simulink model "TVModel_Simulation_21"  (R2021b)
settings: Solver=FixedStepDiscrete  StartTime=0.0  StopTime=250  FixedStep=0.02  MaxStep=0.01  RelTol=1e-3
undefined symbols (not defined in the file or in its folder): MB, TV, TV_OLD
libraries: simulink x22, simulink_extras x14, eeGeneralControl x13, slpidlib x8, fuzblock x4, controlLib x4, cstblocks x3, dspstat3 x2, eeSlidingModeController x1, sharedTrackingLibrary x1
(part 4 of 9)

== system TVModel_Simulation_21/Subsystem/Subsystem1/Torque Distribution/MPC/States Constraints ==
  In Bus Element16 : Inport  PortName=torque_limits  Element=t_limit_negative
  In Bus Element3 : Inport  PortName=torque_limits  Element=t_limit_positive
  In Bus Element6 : Inport  Port=2  PortName=TC_Torque  Element=Regen
  In Bus Element7 : Inport  Port=2  PortName=TC_Torque  Element=Traction
  In Bus Element1 : Inport  Port=3  PortName=dynamics_data
  In Bus Element4 : Inport  Port=4  PortName=slip_ratio
  In Bus Element13 : Inport  Port=5  PortName=brake_signal
  In Bus Element5 : Inport  Port=6  PortName=driver_inputs  Element=brake
  In Bus Element19 : Inport  Port=6  PortName=driver_inputs  Element=throttle
  Bus Element In1 : Inport  Port=7  PortName=slip_angles
  Bus Element In11 : Inport  Port=8  PortName=Fz
  Bus Element In : Inport  Port=9  PortName=epsilon
  Anti reverse wheelspin : Subsystem
  Brake & ESP : Subsystem
  Cross Check : MATLAB Function  TreatAsAtomicUnit=on
  Low YRD : Subsystem
  MATLAB Function : MATLAB Function  TreatAsAtomicUnit=on
  MATLAB Function1 : MATLAB Function  TreatAsAtomicUnit=on
  Min : MinMax  Inputs=3
  Min1 : MinMax  Function=max  Inputs=3
  Tire Bounds : Subsystem
      settings: PortSchema="{\"entries\":[{\"content\":{\"sides\":[{\"content\":{\"connectorIds\":[\"In1\",\"In2\",\"In3\"]},\"type\":\"ConnectorPlacement.EquallySpacedRectSide\",\"uuid\":\"c905e0d5-9d26-4c00-bd7e-07ee0633c160\"},{\"content\":{\"connectorIds\":[\"Out1\",\"Out2\"],\"side\":\"RIGHT\"},\"type\":\"ConnectorPlacement.EquallySpacedRectSide\",\"uuid\":\"37cd4095-0f8c-481f-b8de-23350fc0b3e2\"},{\"content\":{\"connectorIds\":[\"Out3\"],\"side\":\"TOP\"},\"type\":\"ConnectorPlacement.EquallySpacedRectSide\",\"uuid\":\"585cff9f-4d8e-4579-999e-dff949f4791c\"}]},\"type\":\"ConnectorPlacement.EquallySpacedConnector\",\"uuid\":\"48494429-6ae2-4bc0-abe5-17d5f904d891\"}],\"packageUris\":[\"http://schema.mathworks.com/mf0/Connector/R2020b\"],\"version\":\"1.0\"}"
  Unary Minus : UnaryMinus
  lbx : Outport
  ubx : Outport  Port=2
  Out Bus Element2 : Outport  Port=3  PortName=TV_Info  Element=ubx
  Out Bus Element3 : Outport  Port=3  PortName=TV_Info  Element=lbx
  Out Bus Element1 : Outport  Port=3  PortName=TV_Info  Element=Tire_Bounds
  wires:
  In Bus Element19/1 -> Cross Check/5(throttle)
  Bus Element In/1 -> Cross Check/4(epsilon)
  In Bus Element7/1 -> Min/2
  Min1/1 -> Anti reverse wheelspin/1(lbx_in), Low YRD/2(lbx_max)
  Low YRD/1(bounds) -> Cross Check/2(bounds)
  Anti reverse wheelspin/1(lbx_out) -> Cross Check/3(lbx_in), Low YRD/3(lbx_in)
  MATLAB Function1/1(y) -> lbx/1
  MATLAB Function/1(y) -> ubx/1
  In Bus Element16/1 -> Unary Minus/1
  Cross Check/1(ubx_out) -> Out Bus Element2/1, MATLAB Function/1(u)
  Bus Element In1/1 -> Tire Bounds/2(slip_angle)
  Bus Element In11/1 -> Tire Bounds/1(fz)
  Tire Bounds/3(TV_Info) -> Out Bus Element1/1
  In Bus Element1/1 -> Tire Bounds/3(dynamics_data)
  Tire Bounds/1(tire_ubx) -> Min/3
  Tire Bounds/2(tire_lbx) -> Min1/1
  Min/1 -> Brake & ESP/1(ubx_in)
  Brake & ESP/1(ubx_out) -> Cross Check/1(ubx_in), Low YRD/1(ubx_in)
  In Bus Element13/1 -> Brake & ESP/2(brake_signal)
  In Bus Element4/1 -> Anti reverse wheelspin/2(slip_ratio)
  In Bus Element5/1 -> Cross Check/6(brake)
  In Bus Element6/1 -> Min1/3
  In Bus Element3/1 -> Min/1
  Unary Minus/1 -> Min1/2
  Cross Check/2(lbx_out) -> MATLAB Function1/1(u), Out Bus Element3/1

== system TVModel_Simulation_21/Subsystem/Subsystem1/Torque Distribution/MPC/USEFUL STUFFFF ==
  In Bus Element10 : Inport  PortName=front_wheels_steering  Element=single_axis
  Abs : Abs  Commented=on
  Chart : Stateflow chart  Commented=on  TreatAsAtomicUnit=on
  Constant3 : Constant  Commented=on  Value=TV.SIGNALS.SETTINGS.steer_threshold
  Constant5 : Constant  Commented=on  Value=TV.SIGNALS.SETTINGS.steer_relay_amplitude
  Extended Kalman Filter : Subsystem  Commented=on
  Non-Linear Activation : MATLAB Function  Commented=on  TreatAsAtomicUnit=on
  Power Limiter : Subsystem  Commented=on
  Power flag : Subsystem  Commented=on
  Radians to Degrees : simulink_extras/Transformations/Radians to Degrees  Commented=on
  States Selector : Subsystem  Commented=on
  Subsystem : Subsystem  Commented=on
  Subsystem1 : Subsystem  Commented=on
  Yrd 0 When Steering 0 : Subsystem  Commented=on
      mask Display: image('Mask_Icon\On_Off.png'); % Use "Edit Image" on toolstrip to change.
  lbu_dot : Subsystem  Commented=on
  wires:
  Power flag/1(Output) -> ?
  Subsystem/1(Output) -> ?
  Abs/1 -> Chart/1(front_wheels_steering)
  In Bus Element10/1 -> Radians to Degrees/1
  Constant5/1 -> Chart/2(semi_amplitude)
  Radians to Degrees/1 -> Abs/1
  Constant3/1 -> Chart/3(steer_threshold)

== system TVModel_Simulation_21/Subsystem/Subsystem1/Torque Distribution/MPC/Useful Calculations ==
  In Bus Element16 : Inport  PortName=dynamics_data
  In Bus Element1 : Inport  PortName=dynamics_data  Element=omega_wheels
  In Bus Element18 : Inport  Port=2  PortName=front_wheel_angles  Element=different_axis
  Inport : Inport  Port=3
  Abs : Abs
  Gain : Gain  Gain=13.5
  Inport1 : InportShadow  Port=3
  MATLAB Function : MATLAB Function  TreatAsAtomicUnit=on
  MATLAB Function1 : MATLAB Function  TreatAsAtomicUnit=on
  MATLAB Function2 : MATLAB Function  TreatAsAtomicUnit=on
  Power Calculation Post : Subsystem
  Terminator{,1..3} (4 alike) : Terminator
  wires:
  Abs/1 -> MATLAB Function2/2(t)
  Gain/1 -> MATLAB Function2/1(omega)
  In Bus Element1/1 -> Gain/1
  MATLAB Function2/1(y) -> Terminator3/1  "p_MPC"
  MATLAB Function1/2(deltag4) -> Terminator2/1  "deltag4"
  MATLAB Function1/1(deltag3) -> Terminator1/1  "deltag3"
  Inport1/1 -> MATLAB Function/1(T), MATLAB Function1/1(u), Abs/1
  Inport/1 -> Power Calculation Post/2(Motor_Torque)
  In Bus Element18/1 -> MATLAB Function/2(delta)
  MATLAB Function/1(y) -> Terminator/1  "Mz_Real"
  In Bus Element16/1 -> Power Calculation Post/1(dynamics_data)

== system TVModel_Simulation_21/Subsystem/Subsystem1/Torque Distribution/MPC/Weights Generation ==
  In Bus Element1 : Inport  PortName=dynamics_data
  Torque : Inport  Port=2
  Constant : Constant  Value=1e-5*ones(4,1)
  Constant1 : Constant  Value=0  VectorParams1D=off
  Constant2 : Constant  Value=1e-4*ones(4,1)
  Demux : Demux
  Demux1 : Demux
  Efficiency limit : Subsystem  Commented=on
  Gain : Gain  Commented=on  Gain=TV.SIGNALS.SETTINGS.TorqueWeight
  MATLAB Function : MATLAB Function  TreatAsAtomicUnit=on
  Mux : Mux  Inputs=TV.MPC.ny
  r1 : Constant
  vx : Constant  Value=0
  vy : Constant  Value=TV.SIGNALS.SETTINGS.VyWeight
  w : Outport
  Out Bus Element3 : Outport  Port=2  PortName=TV_Info  Element=w
  wires:
  Constant2/1 -> Demux/1
  Efficiency limit/1(efficiency_limit) -> Gain/1
  Constant/1 -> Demux1/1
  Demux1/2 -> Mux/9
  Demux1/4 -> Mux/11
  Demux1/1 -> Mux/8
  Demux1/3 -> Mux/10
  vy/1 -> Mux/2
  vx/1 -> Mux/1
  MATLAB Function/1(y) -> Out Bus Element3/1, w/1
  Demux/1 -> Mux/4
  Demux/2 -> Mux/5
  Demux/4 -> Mux/7
  Demux/3 -> Mux/6
  Torque/1 -> Efficiency limit/1(motor_torque)
  In Bus Element1/1 -> Efficiency limit/2(dynamics_data)
  r1/1 -> Mux/3
  Constant1/1 -> MATLAB Function/2(deltaAxle)
  Mux/1 -> MATLAB Function/1(u)

== system TVModel_Simulation_21/Subsystem/Subsystem1/Torque Distribution/Reference Tracking/YRD_LUT_-1 ==
  front_wheel_angle : Inport
  vx : Inport  Port=2
  Action Port : ActionPort  ActionPortLabel=elseif(u1 ==4)
  Abs : Abs
  Cast3 : DataTypeConversion  Commented=on  OutDataTypeStr=single
  Divide : Product  Inputs=*/
  Divide1 : Product  Inputs=*/
  Divide2 : Product  Inputs=**
  LUT_-3 : Lookup_n-D  BreakpointsForDimension1=TV.LUT.Yrd_LUT.LUT_vectors.delta_vector  BreakpointsForDimension2=TV.LUT.Yrd_LUT.LUT_vectors.v_vector  Table=single(TV.LUT.Yrd_LUT.LUT_neg3.ay_matrix)  InternalRulePriority=Speed  RndMeth=Simplest  InputSameDT=on
      settings: InputPortMap=u0,u1
  Saturation : Saturate  UpperLimit=inf  LowerLimit=3
  yrd : Outport
  wires:
  Divide1/1 -> Divide2/1  "normalized_front_wheel_angle"
  Divide2/1 -> yrd/1  "yrd"
  Saturation/1 -> LUT_-3/2, Divide/2  "vx"
  vx/1 -> Saturation/1
  LUT_-3/1 -> Divide/1  "a"
  Divide/1 -> Divide2/2
  Abs/1 -> LUT_-3/1, Divide1/2  "absolute_front_wheel_angle"
  front_wheel_angle/1 -> Abs/1, Divide1/1

== system TVModel_Simulation_21/Subsystem/Subsystem1/Torque Distribution/Reference Tracking/YRD_LUT_-1.1 ==
  front_wheel_angle : Inport
  vx : Inport  Port=2
  Action Port : ActionPort  ActionPortLabel=elseif(u1 ==3)
  Abs : Abs
  Cast3 : DataTypeConversion  Commented=on  OutDataTypeStr=single
  Divide : Product  Inputs=*/
  Divide1 : Product  Inputs=*/
  Divide2 : Product  Inputs=**
  LUT_-1.5 : Lookup_n-D  BreakpointsForDimension1=TV.LUT.Yrd_LUT.LUT_vectors.delta_vector  BreakpointsForDimension2=TV.LUT.Yrd_LUT.LUT_vectors.v_vector  Table=single(TV.LUT.Yrd_LUT.LUT_neg1_5.ay_matrix)  InternalRulePriority=Speed  RndMeth=Simplest  InputSameDT=on
      settings: InputPortMap=u0,u1
  Saturation : Saturate  UpperLimit=inf  LowerLimit=3
  yrd : Outport
  wires:
  Divide/1 -> Divide2/2
  LUT_-1.5/1 -> Divide/1
  Saturation/1 -> LUT_-1.5/2, Divide/2  "vx"
  Abs/1 -> LUT_-1.5/1, Divide1/2  "absolute_front_wheel_angle"
  Divide2/1 -> yrd/1  "yrd"
  Divide1/1 -> Divide2/1  "normalized_front_wheel_angle"
  vx/1 -> Saturation/1
  front_wheel_angle/1 -> Abs/1, Divide1/1

== system TVModel_Simulation_21/Subsystem/Subsystem1/Torque Distribution/Reference Tracking/YRD_LUT_-1.5 ==
  front_wheel_angle : Inport
  vx : Inport  Port=2
  Action Port : ActionPort  ActionPortLabel=elseif(u1 ==3)
  Abs : Abs
  Cast3 : DataTypeConversion  Commented=on  OutDataTypeStr=single
  Divide : Product  Inputs=*/
  Divide1 : Product  Inputs=*/
  Divide2 : Product  Inputs=**
  LUT_-1.5 : Lookup_n-D  BreakpointsForDimension1=TV.LUT.Yrd_LUT.LUT_vectors.delta_vector  BreakpointsForDimension2=TV.LUT.Yrd_LUT.LUT_vectors.v_vector  Table=single(TV.LUT.Yrd_LUT.LUT_neg1_5.ay_matrix)  InternalRulePriority=Speed  RndMeth=Simplest  InputSameDT=on
      settings: InputPortMap=u0,u1
  Saturation : Saturate  UpperLimit=inf  LowerLimit=3
  yrd : Outport
  wires:
  front_wheel_angle/1 -> Divide1/1, Abs/1
  vx/1 -> Saturation/1
  Divide1/1 -> Divide2/1  "normalized_front_wheel_angle"
  Divide2/1 -> yrd/1  "yrd"
  Abs/1 -> Divide1/2, LUT_-1.5/1  "absolute_front_wheel_angle"
  Saturation/1 -> Divide/2, LUT_-1.5/2  "vx"
  LUT_-1.5/1 -> Divide/1
  Divide/1 -> Divide2/2

== system TVModel_Simulation_21/Subsystem/Subsystem1/Torque Distribution/Reference Tracking/YRD_LUT_-3 ==
  front_wheel_angle : Inport
  vx : Inport  Port=2
  Action Port : ActionPort  ActionPortLabel=elseif(u1 ==4)
  Abs : Abs
  Cast3 : DataTypeConversion  Commented=on  OutDataTypeStr=single
  Divide : Product  Inputs=*/
  Divide1 : Product  Inputs=*/
  Divide2 : Product  Inputs=**
  LUT_-3 : Lookup_n-D  BreakpointsForDimension1=TV.LUT.Yrd_LUT.LUT_vectors.delta_vector  BreakpointsForDimension2=TV.LUT.Yrd_LUT.LUT_vectors.v_vector  Table=single(TV.LUT.Yrd_LUT.LUT_neg3.ay_matrix)  InternalRulePriority=Speed  RndMeth=Simplest  InputSameDT=on
      settings: InputPortMap=u0,u1
  Saturation : Saturate  UpperLimit=inf  LowerLimit=3
  yrd : Outport
  wires:
  front_wheel_angle/1 -> Divide1/1, Abs/1
  Abs/1 -> Divide1/2, LUT_-3/1  "absolute_front_wheel_angle"
  Divide/1 -> Divide2/2
  LUT_-3/1 -> Divide/1  "a"
  vx/1 -> Saturation/1
  Saturation/1 -> Divide/2, LUT_-3/2  "vx"
  Divide2/1 -> yrd/1  "yrd"
  Divide1/1 -> Divide2/1  "normalized_front_wheel_angle"

== system TVModel_Simulation_21/Subsystem/Subsystem1/Torque Distribution/Reference Tracking/YRD_LUT_0 ==
  front_wheel_angle : Inport
  vx : Inport  Port=2
  Action Port : ActionPort  ActionPortLabel=elseif(u1 ==2)
  Abs : Abs
  Cast : DataTypeConversion  Commented=on  OutDataTypeStr=single
  Divide : Product  Inputs=*/
  Divide1 : Product  Inputs=*/
  Divide2 : Product  Inputs=**
  LUT_0 : Lookup_n-D  BreakpointsForDimension1=TV.LUT.Yrd_LUT.LUT_vectors.delta_vector  BreakpointsForDimension2=TV.LUT.Yrd_LUT.LUT_vectors.v_vector  Table=single(TV.LUT.Yrd_LUT.LUT_0.ay_matrix)  InternalRulePriority=Speed  RndMeth=Simplest  InputSameDT=on
      settings: InputPortMap=u0,u1
  Saturation : Saturate  UpperLimit=inf  LowerLimit=3
  yrd : Outport
  wires:
  front_wheel_angle/1 -> Divide1/1, Abs/1
  Saturation/1 -> Divide/2, LUT_0/2  "vx"
  Abs/1 -> Divide1/2, LUT_0/1  "absolute_front_wheel_angle"
  Divide2/1 -> yrd/1  "yrd"
  vx/1 -> Saturation/1
  Divide/1 -> Divide2/2
  Divide1/1 -> Divide2/1  "normalized_front_wheel_angle"
  LUT_0/1 -> Divide/1

== system TVModel_Simulation_21/Subsystem/Subsystem1/Torque Distribution/Reference Tracking/YRD_LUT_1 ==
  front_wheel_angle : Inport
  vx : Inport  Port=2
  Action Port : ActionPort  ActionPortLabel=if(u1 == 1)
  Abs : Abs
  Cast3 : DataTypeConversion  Commented=on  OutDataTypeStr=single
  Divide : Product  Inputs=*/
  Divide1 : Product  Inputs=*/
  Divide2 : Product  Inputs=**
  LUT_1 : Lookup_n-D  BreakpointsForDimension1=TV.LUT.Yrd_LUT.LUT_vectors.delta_vector  BreakpointsForDimension2=TV.LUT.Yrd_LUT.LUT_vectors.v_vector  Table=single(TV.LUT.Yrd_LUT.LUT_1.ay_matrix)  InternalRulePriority=Speed  RndMeth=Simplest  InputSameDT=on
      settings: InputPortMap=u0,u1
  Saturation : Saturate  UpperLimit=inf  LowerLimit=3
  yrd : Outport
  wires:
  front_wheel_angle/1 -> Divide1/1, Abs/1
  LUT_1/1 -> Divide/1
  vx/1 -> Saturation/1
  Divide1/1 -> Divide2/1  "normalized_front_wheel_angle"
  Divide2/1 -> yrd/1  "yrd"
  Abs/1 -> Divide1/2, LUT_1/1  "absolute_front_wheel_angle"
  Saturation/1 -> Divide/2, LUT_1/2  "vx"
  Divide/1 -> Divide2/2

== system TVModel_Simulation_21/Subsystem/Subsystem1/Torque Distribution/Reference Tracking/YRD_LUT_2 ==
  front_wheel_angle : Inport
  vx : Inport  Port=2
  Action Port : ActionPort  ActionPortLabel=elseif(u1 ==2)
  Abs : Abs
  Cast : DataTypeConversion  Commented=on  OutDataTypeStr=single
  Divide : Product  Inputs=*/
  Divide1 : Product  Inputs=*/
  Divide2 : Product  Inputs=**
  LUT_0 : Lookup_n-D  BreakpointsForDimension1=TV.LUT.Yrd_LUT.LUT_vectors.delta_vector  BreakpointsForDimension2=TV.LUT.Yrd_LUT.LUT_vectors.v_vector  Table=single(TV.LUT.Yrd_LUT.LUT_0.ay_matrix)  InternalRulePriority=Speed  RndMeth=Simplest  InputSameDT=on
      settings: InputPortMap=u0,u1
  Saturation : Saturate  UpperLimit=inf  LowerLimit=3
  yrd : Outport
  wires:
  LUT_0/1 -> Divide/1
  Divide1/1 -> Divide2/1  "normalized_front_wheel_angle"
  Divide/1 -> Divide2/2
  vx/1 -> Saturation/1
  Divide2/1 -> yrd/1  "yrd"
  Abs/1 -> LUT_0/1, Divide1/2  "absolute_front_wheel_angle"
  Saturation/1 -> LUT_0/2, Divide/2  "vx"
  front_wheel_angle/1 -> Abs/1, Divide1/1

== system TVModel_Simulation_21/Subsystem/Subsystem1/Torque Distribution/Reference Tracking/YRD_LUT_3 ==
  front_wheel_angle : Inport
  vx : Inport  Port=2
  Action Port : ActionPort  ActionPortLabel=if(u1 == 1)
  Abs : Abs
  Cast3 : DataTypeConversion  Commented=on  OutDataTypeStr=single
  Divide : Product  Inputs=*/
  Divide1 : Product  Inputs=*/
  Divide2 : Product  Inputs=**
  LUT_1 : Lookup_n-D  BreakpointsForDimension1=TV.LUT.Yrd_LUT.LUT_vectors.delta_vector  BreakpointsForDimension2=TV.LUT.Yrd_LUT.LUT_vectors.v_vector  Table=single(TV.LUT.Yrd_LUT.LUT_1.ay_matrix)  InternalRulePriority=Speed  RndMeth=Simplest  InputSameDT=on
      settings: InputPortMap=u0,u1
  Saturation : Saturate  UpperLimit=inf  LowerLimit=3
  yrd : Outport
  wires:
  Divide/1 -> Divide2/2
  Saturation/1 -> LUT_1/2, Divide/2  "vx"
  Abs/1 -> LUT_1/1, Divide1/2  "absolute_front_wheel_angle"
  Divide2/1 -> yrd/1  "yrd"
  Divide1/1 -> Divide2/1  "normalized_front_wheel_angle"
  vx/1 -> Saturation/1
  LUT_1/1 -> Divide/1
  front_wheel_angle/1 -> Abs/1, Divide1/1

== system TVModel_Simulation_21/Subsystem/Subsystem1/Torque Limits/Torque Limits Positive/Torque_Curve ==
  omega_wheels : Inport
  voltage [ID380] : Inport  Port=2
  torque_map : Inport  Port=3
  2-D Lookup Table : Lookup_n-D  BreakpointsForDimension1=TV.LV.TORQUE.T_lim_pos.breakpoints1  BreakpointsForDimension2=TV.LV.TORQUE.T_lim_pos.breakpoints2  Table=TV.LV.TORQUE.T_lim_pos.table_data  ExtrapMethod=Clip  InternalRulePriority=Speed  OutDataTypeStr=double  RndMeth=Simplest  InputSameDT=on
      settings: InputPortMap=u0,u1
  Constant : Constant  Value=0
  Constant1 : Constant  Value=TV.LV.TORQUE.T_peak_motor
  Constant2 : Constant  Value=TV.LV.TORQUE.T_nominal_motor
  Gain : Gain  Gain=TV.LV.TORQUE.T_nominal_motor/1000
  Gain4 : Gain  Gain=TV.CAR.Tau*60/(2*pi)
  Low-Pass Filter (Discrete or Continuous) : eeGeneralControl/Low-Pass Filter (Discrete or Continuous)  K=1  T=1/4/pi  B=inf  A=-inf  init_option=Inherited from block input  x0=0  Ts=TV.MPC.T/TV.MPC.N
  Multiport Switch : MultiPortSwitch  DataPortOrder=Specify indices  DataPortIndices={TV.LV.TORQUE.T_peak_setting,TV.LV.TORQUE.T_nominal_setting}  DiagnosticForDefault=None
  Saturation Dynamic : simulink/Discontinuities/Saturation Dynamic  OutMin=[]  OutMax=[]  OutDataTypeStr=Inherit: Same as second input  OutDataType=fixdt(1, 16)  OutScaling=2^-10  DoSatur=off
  Saturation1 : Saturate  UpperLimit=+inf  LowerLimit=0
  max_torque_available : Outport
  wires:
  Low-Pass Filter (Discrete or Continuous)/1 -> Saturation Dynamic/2
  omega_wheels/1 -> Gain4/1
  Constant/1 -> Saturation Dynamic/3
  torque_map/1 -> Multiport Switch/1
  Constant1/1 -> Multiport Switch/2
  Constant2/1 -> Multiport Switch/3
  Multiport Switch/1 -> Saturation Dynamic/1  "torque map selected"
  Saturation1/1 -> 2-D Lookup Table/1
  voltage [ID380]/1 -> 2-D Lookup Table/2
  Gain/1 -> Low-Pass Filter (Discrete or Continuous)/1
  2-D Lookup Table/1 -> Gain/1
  Gain4/1 -> Saturation1/1  "RPM_Motors"
  Saturation Dynamic/1 -> max_torque_available/1

== system TVModel_Simulation_21/Subsystem/Subsystem1/Torque Limits/Torque Limits Regen/Torque_Curve ==
  omega_wheels : Inport
  voltage [ID380] : Inport  Port=2
  torque_map : Inport  Port=3
  2-D Lookup Table : Lookup_n-D  BreakpointsForDimension1=TV.LV.TORQUE.T_lim_pos.breakpoints1  BreakpointsForDimension2=TV.LV.TORQUE.T_lim_pos.breakpoints2  Table=TV.LV.TORQUE.T_lim_pos.table_data  ExtrapMethod=Clip  InternalRulePriority=Speed  OutDataTypeStr=double  RndMeth=Simplest  InputSameDT=on
      settings: InputPortMap=u0,u1
  Constant : Constant  Value=0
  Constant1 : Constant  Value=TV.LV.TORQUE.T_peak_motor
  Constant2 : Constant  Value=TV.LV.TORQUE.T_nominal_motor
  Gain : Gain  Gain=TV.LV.TORQUE.T_nominal_motor/1000
  Gain4 : Gain  Gain=TV.CAR.Tau*60/(2*pi)
  Low-Pass Filter (Discrete or Continuous) : eeGeneralControl/Low-Pass Filter (Discrete or Continuous)  K=1  T=1/4/pi  B=inf  A=-inf  init_option=Inherited from block input  x0=0  Ts=TV.MPC.T/TV.MPC.N
  Multiport Switch : MultiPortSwitch  DataPortOrder=Specify indices  DataPortIndices={TV.LV.TORQUE.T_peak_setting,TV.LV.TORQUE.T_nominal_setting}  DiagnosticForDefault=None
  Saturation Dynamic : simulink/Discontinuities/Saturation Dynamic  OutMin=[]  OutMax=[]  OutDataTypeStr=Inherit: Same as second input  OutDataType=fixdt(1, 16)  OutScaling=2^-10  DoSatur=off
  Saturation1 : Saturate  UpperLimit=+inf  LowerLimit=0
  max_torque_available : Outport
  wires:
  Low-Pass Filter (Discrete or Continuous)/1 -> Saturation Dynamic/2
  omega_wheels/1 -> Gain4/1
  Constant/1 -> Saturation Dynamic/3
  torque_map/1 -> Multiport Switch/1
  Constant1/1 -> Multiport Switch/2
  Constant2/1 -> Multiport Switch/3
  Multiport Switch/1 -> Saturation Dynamic/1  "torque map selected"
  Saturation1/1 -> 2-D Lookup Table/1
  voltage [ID380]/1 -> 2-D Lookup Table/2
  Gain/1 -> Low-Pass Filter (Discrete or Continuous)/1
  2-D Lookup Table/1 -> Gain/1
  Gain4/1 -> Saturation1/1  "RPM_Motors"
  Saturation Dynamic/1 -> max_torque_available/1

== system TVModel_Simulation_21/Subsystem/Subsystem1/Slip Control/Traction Control/ABS/Load Transfer Calculation1 ==
  In Bus Element : Inport  PortName=dynamics_data
  Fz FL : Subsystem
  Fz FR : Subsystem
  Fz RL : Subsystem
  Fz RR : Subsystem
  Mux : Mux
  Fz [4x1] : Outport
  wires:
  In Bus Element/1 -> Fz FL/1(dynamics_data), Fz FR/1(dynamics_data), Fz RL/1(dynamics_data), Fz RR/1(dynamics_data)
  Fz FL/1(TV_Info) -> Mux/1  "Fz_FL"
  Fz FR/1(TV_Info) -> Mux/2  "Fz_FR"
  Fz RL/1(TV_Info) -> Mux/3  "Fz_RL"
  Fz RR/1(TV_Info) -> Mux/4  "Fz_RR"
  Mux/1 -> Fz [4x1]/1

== system TVModel_Simulation_21/Subsystem/Subsystem1/Slip Control/Traction Control/ABS/Subsystem ==
  Inport : Inport
  Inport1 : Inport  Port=2
  Chart : Stateflow chart  TreatAsAtomicUnit=on
  Chart1 : Stateflow chart  TreatAsAtomicUnit=on
  Chart2 : Stateflow chart  TreatAsAtomicUnit=on
  Chart3 : Stateflow chart  TreatAsAtomicUnit=on
  Demux : Demux
  Demux1 : Demux
  Mux : Mux
  Output : Outport
  wires:
  Demux/1 -> Chart/2(epsilon)
  Demux/2 -> Chart1/2(epsilon)
  Demux/3 -> Chart2/2(epsilon)
  Demux/4 -> Chart3/2(epsilon)
  Demux1/4 -> Chart3/1(T_ff)
  Demux1/3 -> Chart2/1(T_ff)
  Demux1/2 -> Chart1/1(T_ff)
  Demux1/1 -> Chart/1(T_ff)
  Inport/1 -> Demux1/1
  Inport1/1 -> Demux/1
  Mux/1 -> Output/1  "TC_output"
  Chart3/1(TC_max) -> Mux/4  "TC_output"
  Chart2/1(TC_max) -> Mux/3  "TC_output"
  Chart1/1(TC_max) -> Mux/2  "TC_output"
  Chart/1(TC_max) -> Mux/1  "TC_output"

== system TVModel_Simulation_21/Subsystem/Subsystem1/Slip Control/Traction Control/Load Transfer calculation/Fz FL ==
  In Bus Element : Inport  PortName=dynamics_data  Element=ay
  In Bus Element1 : Inport  PortName=dynamics_data  Element=vx
  In Bus Element2 : Inport  PortName=dynamics_data  Element=ax
  Drag moment : Gain  Gain=0.5*TV.CAR.rho*TV.CAR.CdA*TV.CAR.hcop/TV.CAR.wb*0.5
  Lateral Load Transfer : Gain  Gain=TV.CAR.m/TV.CAR.tf*TV.CAR.hcog*0.5*0.5
  Lift Force : Gain  Gain=0.5*TV.CAR.rho*TV.CAR.ClA*(1-TV.CAR.xcop/TV.CAR.wb)*0.5
  Longitudinal Load Transfer : Gain  Gain=TV.CAR.m/TV.CAR.wb*TV.CAR.hcog*0.5
  Square1 : Math  Operator=square  SaturateOnIntegerOverflow=on
  Square2 : Math  Operator=square  SaturateOnIntegerOverflow=on
  Static Load Front : Constant  Value=TV.CAR.Fzf
  Subtract : Sum  Inputs=+++-+
  Unary Minus : UnaryMinus
  Unary Minus1 : UnaryMinus
  TV_Info : Outport
  wires:
  Unary Minus1/1 -> Longitudinal Load Transfer/1
  Unary Minus/1 -> Lateral Load Transfer/1
  In Bus Element/1 -> Unary Minus/1
  Subtract/1 -> TV_Info/1
  Drag moment/1 -> Subtract/4
  Static Load Front/1 -> Subtract/1
  Square1/1 -> Lift Force/1
  Lateral Load Transfer/1 -> Subtract/2
  Longitudinal Load Transfer/1 -> Subtract/5
  In Bus Element2/1 -> Unary Minus1/1
  Square2/1 -> Drag moment/1
  In Bus Element1/1 -> Square2/1, Square1/1
  Lift Force/1 -> Subtract/3

== system TVModel_Simulation_21/Subsystem/Subsystem1/Slip Control/Traction Control/Load Transfer calculation/Fz FR ==
  In Bus Element : Inport  PortName=dynamics_data  Element=ay
  In Bus Element1 : Inport  PortName=dynamics_data  Element=vx
  In Bus Element2 : Inport  PortName=dynamics_data  Element=ax
  Drag moment : Gain  Gain=0.5*TV.CAR.rho*TV.CAR.CdA*TV.CAR.hcop/TV.CAR.wb*0.5
  Lateral Load Transfer : Gain  Gain=TV.CAR.m/TV.CAR.tf*TV.CAR.hcog*0.5*0.5
  Lift Force : Gain  Gain=0.5*TV.CAR.rho*TV.CAR.ClA*(1 - TV.CAR.xcop/TV.CAR.wb)*0.5
  Longitudinal Load Transfer : Gain  Gain=TV.CAR.m/TV.CAR.wb*TV.CAR.hcog*0.5
  Square1 : Math  Operator=square  SaturateOnIntegerOverflow=on
  Square2 : Math  Operator=square  SaturateOnIntegerOverflow=on
  Static Load Front : Constant  Value=TV.CAR.Fzf
  Subtract : Sum  Inputs=+-+-+
  Unary Minus : UnaryMinus
  Unary Minus1 : UnaryMinus
  TV_Info : Outport
  wires:
  Unary Minus1/1 -> Longitudinal Load Transfer/1
  Unary Minus/1 -> Lateral Load Transfer/1
  Subtract/1 -> TV_Info/1
  Drag moment/1 -> Subtract/4
  In Bus Element/1 -> Unary Minus/1
  In Bus Element1/1 -> Square1/1, Square2/1
  Static Load Front/1 -> Subtract/1
  Square1/1 -> Lift Force/1
  Lateral Load Transfer/1 -> Subtract/2
  Longitudinal Load Transfer/1 -> Subtract/5
  In Bus Element2/1 -> Unary Minus1/1
  Lift Force/1 -> Subtract/3
  Square2/1 -> Drag moment/1

== system TVModel_Simulation_21/Subsystem/Subsystem1/Slip Control/Traction Control/Load Transfer calculation/Fz RL ==
  In Bus Element : Inport  PortName=dynamics_data  Element=ay
  In Bus Element1 : Inport  PortName=dynamics_data  Element=vx
  In Bus Element2 : Inport  PortName=dynamics_data  Element=ax
  Drag moment : Gain  Gain=0.5*TV.CAR.rho*TV.CAR.CdA*TV.CAR.hcop/TV.CAR.wb*0.5
  Lateral Load Transfer : Gain  Gain=TV.CAR.m/TV.CAR.tr*TV.CAR.hcog*0.5*0.5
  Lift Force : Gain  Gain=0.5*TV.CAR.rho*TV.CAR.ClA*(TV.CAR.xcop/TV.CAR.wb)*0.5
  Longitudinal Load Transfer : Gain  Gain=TV.CAR.m/TV.CAR.wb*TV.CAR.hcog*0.5
  Square1 : Math  Operator=square  SaturateOnIntegerOverflow=on
  Square2 : Math  Operator=square  SaturateOnIntegerOverflow=on
  Static Load Front : Constant  Value=TV.CAR.Fzr
  Subtract : Sum  Inputs=++++-
  Unary Minus : UnaryMinus
  Unary Minus1 : UnaryMinus
  TV_Info : Outport
  wires:
  Unary Minus1/1 -> Longitudinal Load Transfer/1
  Unary Minus/1 -> Lateral Load Transfer/1
  Subtract/1 -> TV_Info/1
  Drag moment/1 -> Subtract/4
  In Bus Element/1 -> Unary Minus/1
  Static Load Front/1 -> Subtract/1
  Square1/1 -> Lift Force/1
  Lateral Load Transfer/1 -> Subtract/2
  Longitudinal Load Transfer/1 -> Subtract/5
  In Bus Element2/1 -> Unary Minus1/1
  Lift Force/1 -> Subtract/3
  Square2/1 -> Drag moment/1
  In Bus Element1/1 -> Square2/1, Square1/1

== system TVModel_Simulation_21/Subsystem/Subsystem1/Slip Control/Traction Control/Load Transfer calculation/Fz RR ==
  In Bus Element : Inport  PortName=dynamics_data  Element=ay
  In Bus Element1 : Inport  PortName=dynamics_data  Element=vx
  In Bus Element2 : Inport  PortName=dynamics_data  Element=ax
  Drag moment : Gain  Gain=0.5*TV.CAR.rho*TV.CAR.CdA*TV.CAR.hcop/TV.CAR.wb*0.5
  Lateral Load Transfer : Gain  Gain=TV.CAR.m/TV.CAR.tr*TV.CAR.hcog*0.5*0.5
  Lift Force : Gain  Gain=0.5*TV.CAR.rho*TV.CAR.ClA*(TV.CAR.xcop/TV.CAR.wb)*0.5
  Longitudinal Load Transfer : Gain  Gain=TV.CAR.m/TV.CAR.wb*TV.CAR.hcog*0.5
  Square1 : Math  Operator=square  SaturateOnIntegerOverflow=on
  Square2 : Math  Operator=square  SaturateOnIntegerOverflow=on
  Static Load Front : Constant  Value=TV.CAR.Fzr
  Subtract : Sum  Inputs=+-++-
  Unary Minus : UnaryMinus
  Unary Minus1 : UnaryMinus
  TV_Info : Outport
  wires:
  Unary Minus1/1 -> Longitudinal Load Transfer/1
  Unary Minus/1 -> Lateral Load Transfer/1
  Subtract/1 -> TV_Info/1
  Drag moment/1 -> Subtract/4
  In Bus Element/1 -> Unary Minus/1
  In Bus Element1/1 -> Square1/1, Square2/1
  Static Load Front/1 -> Subtract/1
  Square1/1 -> Lift Force/1
  Lateral Load Transfer/1 -> Subtract/2
  Longitudinal Load Transfer/1 -> Subtract/5
  In Bus Element2/1 -> Unary Minus1/1
  Lift Force/1 -> Subtract/3
  Square2/1 -> Drag moment/1

== system TVModel_Simulation_21/Subsystem/Subsystem1/Slip Control/Traction Control/S-R Flip Flops/Subsystem ==
  In1 : Inport
  In2 : Inport  Port=2
  Demux : Demux
  Demux1 : Demux
  Mux : Mux
  S-R Flip-Flop{,1..3} (4 alike) : simulink_extras/Flip Flops/S-R Flip-Flop  initial_condition=0
  Out1 : Outport
  wires:
  Demux1/1 -> S-R Flip-Flop/2
  Demux1/2 -> S-R Flip-Flop1/2
  Demux/4 -> S-R Flip-Flop3/1
  Demux/1 -> S-R Flip-Flop/1
  In1/1 -> Demux/1
  Demux1/3 -> S-R Flip-Flop2/2
  Demux/2 -> S-R Flip-Flop1/1
  Demux1/4 -> S-R Flip-Flop3/2
  S-R Flip-Flop2/1 -> Mux/3
  Demux/3 -> S-R Flip-Flop2/1
  S-R Flip-Flop3/1 -> Mux/4
  In2/1 -> Demux1/1
  Mux/1 -> Out1/1
  S-R Flip-Flop1/1 -> Mux/2
  S-R Flip-Flop/1 -> Mux/1

== system TVModel_Simulation_21/Subsystem/Subsystem1/Slip Control/Traction Control/Slip Control/ABS ==
  eps_target : Inport
  eps : Inport  Port=2
  Reset Signal : Inport  Port=3
  T_actual : Inport  Port=4  PortDimensions=4
  T_limit : Inport  Port=5
  RTD_flag : Inport  Port=6
  Activation logic : Stateflow chart  TreatAsAtomicUnit=on
  Constant : Constant  Value=0.01
  Constant1 : Constant  Value=57/2
  Constant2 : Constant  Value=2845/3
  Constant3 : Constant  Value=0.1
  Constant4 : Constant  Value=-21
  Constant5 : Constant  Value=0.6
  Gain : Gain  Gain=-1
  Minus : Sum  Inputs=+-
  PID Controller5 : slpidlib/PID Controller  Controller=PI  Form=Parallel  TimeDomain=Discrete-time  UseExternalTs=off  SampleTime=0.02  IntegratorMethod=Forward Euler  FilterMethod=Forward Euler  ControllerParametersSource=external  P=57  I=2845  D=0  UseFilter=off  N=63.8249907657072  TunerSelectOption=Transfer Function Based (PID Tuner App)  InitialConditionSource=internal  InitialConditionForIntegrator=0  InitialConditionForFilter=0  DifferentiatorICPrevScaledInput=0  ExternalReset=rising  TrackingMode=on  Kt=TV_OLD.LV.GEN.slipKt  LimitOutput=on  SatLimitsSource=external  UpperSaturationLimit=0  LowerSaturationLimit=-TV_OLD.LV.Tpeak  LinearizeAsGain=on  AntiWindupMode=clamping  Kb=1  POutMin=[]  POutMax=[]  IOutMin=[]  IOutMax=[]  DOutMin=[]  DOutMax=[]  NOutMin=[]  NOutMax=[]  SumOutMin=[]  SumOutMax=[]  SaturationOutMin=[]  SaturationOutMax=[]  PParamMin=[]  PParamMax=[]  IParamMin=[]  IParamMax=[]  DParamMin=[]  DParamMax=[]  NParamMin=[]  NParamMax=[]  KbParamMin=[]  KbParamMax=[]  KtParamMin=[]  KtParamMax=[]  KbOutMin=[]  KbOutMax=[]  KtOutMin=[]  KtOutMax=[]  IntegratorOutMin=[]  IntegratorOutMax=[]  FilterOutMin=[]  FilterOutMax=[]  SumI1OutMin=[]  SumI1OutMax=[]  SumI2OutMin=[]  SumI2OutMax=[]  SumI3OutMin=[]  SumI3OutMax=[]  SumI4OutMin=[]  SumI4OutMax=[]  SumDOutMin=[]  SumDOutMax=[]  DifferentiatorOutMin=[]  DifferentiatorOutMax=[]  FilterDiffOutCoefMin=[]  FilterDiffOutCoefMax=[]  ReciprocalOutMin=[]  ReciprocalOutMax=[]  SumDenOutMin=[]  SumDenOutMax=[]  SumNumOutMin=[]  SumNumOutMax=[]  DivideOutMin=[]  DivideOutMax=[]  UdiffTsProdOutMin=[]  UdiffTsProdOutMax=[]  NTsProdOutMin=[]  NTsProdOutMax=[]  UintegralTsProdOutMin=[]  UintegralTsProdOutMax=[]  UngainTsProdOutMin=[]  UngainTsProdOutMax=[]  IntegratorContinuousStateAttributes=''  IntegratorStateMustResolveToSignalObject=off  IntegratorRTWStateStorageClass=Auto  FilterContinuousStateAttributes=''  FilterStateMustResolveToSignalObject=off  FilterRTWStateStorageClass=Auto  ParallelPVariant=ExternalParameters  IdealPVariant=Disabled  IVariant=ExternalParameters  DVariant=Disabled  IntegratorVariant=Discrete  SatVariant=External  AWVariant=DiscClampingParallel  PCopyVariant=Disabled  TRVariant=Enabled  FdbkBlocksVariant=Forward  IdealPFdbkVariant=Disabled  SatFdbkVariant=Disabled  DerivativeFilterVariant=Disabled  NVariant=Disabled  NCopyVariant=Disabled_SignalSpec  FilterICVariant=Disabled  IntegratorICVariant=InternalICs  ExternalResetVariant=ExternalReset  TRSumVariant=TrackingMode  SumFdbkVariant=Disabled  SumVariant=Sum_PI  TsampFilterVariant=InternalTs  TsampNgainVariant=Passthrough  TsampIntegralVariant=Passthrough  ExternalSaturationOutDataTypeStr=Inherit: Same as second input
  Unit Delay : UnitDelay  InitialCondition=zeros(4,1)  SampleTime=-1  HasFrameUpgradeWarning=on
  Tmin : Outport
  wires:
  Constant2/1 -> PID Controller5/3
  Constant1/1 -> PID Controller5/2
  [ResetSignal] -> Activation logic/6(TC_flag)
  [ResetSignal] -> PID Controller5/4
  Reset Signal/1 -> [ResetSignal]
  [eps] -> Activation logic/3(eps)
  [eps] -> Minus/2
  eps/1 -> [eps]
  [eps_target] -> Activation logic/2(epsTarget)
  eps_target/1 -> [eps_target]
  Minus/1 -> PID Controller5/1
  Activation logic/1(T_min) -> Tmin/1, Unit Delay/1, PID Controller5/7
  T_actual/1 -> Activation logic/4(T_actual)
  Unit Delay/1 -> Activation logic/7(Tmin_old)
  [eps_target] -> Minus/1
  PID Controller5/1 -> Activation logic/1(Tmin_PI)  "Tmin_PI"
  T_limit/1 -> Activation logic/5(T_limit)
  Constant/1 -> Activation logic/8(slipNoise)
  Constant3/1 -> Gain/1
  Gain/1 -> PID Controller5/5
  Constant4/1 -> PID Controller5/6
  Constant5/1 -> Activation logic/9(slipDeactPerc)
  RTD_flag/1 -> Activation logic/10(RTD_flag)

== system TVModel_Simulation_21/Subsystem/Subsystem1/Slip Control/Traction Control/Slip Control/Reset ABS ==
  V : Inport
  throttle : Inport  Port=2
  brake : Inport  Port=3
  TC_setting : Inport  Port=4
  RTD : Inport  Port=5
  AND : Logic  Inputs=3  IconShape=distinctive  AllPortsSameDT=off  OutDataTypeStr=boolean
  Constant : Constant  Value=0
  Constant1 : Constant  Value=0
  Constant2 : Constant  Value=3
  Data Store Read1 : DataStoreRead  Commented=on  DataStoreName=thresholds  DataStoreElements=thresholds.THROTTLE_RELAY_AMP#thresholds.THROTTLE_NOISE#thresholds.BRAKE_RELAY_AMP#thresholds.BRAKE_NOISE  IndexOptions=Index vector (dialog)  Indices=1  OutputSizes=1
  NOT : Logic  Commented=on  Operator=NOT  IconShape=distinctive  AllPortsSameDT=off  OutDataTypeStr=boolean
  Relational Operator : RelationalOperator  Operator=>  OutDataTypeStr=boolean  RndMeth=Simplest
  Relational Operator3 : RelationalOperator  Operator=>  OutDataTypeStr=boolean  RndMeth=Simplest
  Relational Operator4 : RelationalOperator  Operator=>  OutDataTypeStr=boolean  RndMeth=Simplest
  Variable Amplitude Relay : controlLib/Variable Amplitude Relay  Commented=on  SystemSampleTime=-1  VariantActivationTime=update diagram  Latency=0  AutoFrameSizeCalculation=off
      settings: SourceProductName=VCU Library
  Variable Amplitude Relay1 : controlLib/Variable Amplitude Relay  Commented=on  SystemSampleTime=-1  VariantActivationTime=update diagram  Latency=0  AutoFrameSizeCalculation=off
      settings: SourceProductName=VCU Library
  resetSignal : Outport
  wires:
  Variable Amplitude Relay/1 -> NOT/1
  brake/1 -> Variable Amplitude Relay/3
  throttle/1 -> Variable Amplitude Relay1/3
  Data Store Read1/2 -> Variable Amplitude Relay1/2
  Data Store Read1/3 -> Variable Amplitude Relay/1
  Data Store Read1/4 -> Variable Amplitude Relay/2
  AND/1 -> resetSignal/1
  Relational Operator4/1 -> AND/3
  Relational Operator3/1 -> AND/2
  Relational Operator/1 -> AND/1
  RTD/1 -> Relational Operator4/1
  Constant1/1 -> Relational Operator4/2
  Constant/1 -> Relational Operator3/2
  TC_setting/1 -> Relational Operator3/1
  Data Store Read1/1 -> Variable Amplitude Relay1/1
  V/1 -> Relational Operator/1
  Constant2/1 -> Relational Operator/2

== system TVModel_Simulation_21/Subsystem/Subsystem1/Slip Control/Traction Control/Slip Control/Reset TC ==
  V : Inport
  throttle : Inport  Port=2
  brake : Inport  Port=3
  TC_setting : Inport  Port=4
  RTD : Inport  Port=5
  AND : Logic  Inputs=5  IconShape=distinctive  AllPortsSameDT=off  OutDataTypeStr=boolean
  Constant : Constant  Value=0
  Constant1 : Constant  Value=0
  Constant2 : Constant  Value=3
  Constant3 : Constant  Value=0.01
  Constant4 : Constant  Value=0.05
  Constant5 : Constant  Value=0.01
  Constant6 : Constant  Value=0.1
  NOT : Logic  Operator=NOT  IconShape=distinctive  AllPortsSameDT=off  OutDataTypeStr=boolean
  Relational Operator : RelationalOperator  Operator=>  OutDataTypeStr=boolean  RndMeth=Simplest
  Relational Operator3 : RelationalOperator  Operator=>  OutDataTypeStr=boolean  RndMeth=Simplest
  Relational Operator4 : RelationalOperator  Operator=>  OutDataTypeStr=boolean  RndMeth=Simplest
  Variable Amplitude Relay : controlLib/Variable Amplitude Relay  SystemSampleTime=-1  VariantActivationTime=update diagram  Latency=0  AutoFrameSizeCalculation=off
      settings: SourceProductName=VCU Library
  Variable Amplitude Relay1 : controlLib/Variable Amplitude Relay  SystemSampleTime=-1  VariantActivationTime=update diagram  Latency=0  AutoFrameSizeCalculation=off
      settings: SourceProductName=VCU Library
  resetSignal : Outport
  wires:
  Constant2/1 -> Relational Operator/2
  V/1 -> Relational Operator/1
  Constant3/1 -> Variable Amplitude Relay1/1
  TC_setting/1 -> Relational Operator3/1
  Constant/1 -> Relational Operator3/2
  Constant1/1 -> Relational Operator4/2
  RTD/1 -> Relational Operator4/1
  Relational Operator/1 -> AND/1
  Variable Amplitude Relay1/1 -> AND/2
  NOT/1 -> AND/3
  Relational Operator3/1 -> AND/4
  Relational Operator4/1 -> AND/5
  AND/1 -> resetSignal/1
  Constant6/1 -> Variable Amplitude Relay/2
  Constant5/1 -> Variable Amplitude Relay/1
  Constant4/1 -> Variable Amplitude Relay1/2
  throttle/1 -> Variable Amplitude Relay1/3
  brake/1 -> Variable Amplitude Relay/3
  Variable Amplitude Relay/1 -> NOT/1

== system TVModel_Simulation_21/Subsystem/Subsystem1/Slip Control/Traction Control/Slip Control/Slip computation ==
  <Vx> : Inport
  <Vy> : Inport  Port=2
  <Yaw Rate> : Inport  Port=3
  <deltaL> : Inport  Port=4
  <deltaR> : Inport  Port=5
  Constant : Constant  Value=3
  Constant1 : Constant  Value=1.53/2
  Constant2 : Constant  Value=1.27
  MATLAB Function2 : MATLAB Function  TreatAsAtomicUnit=on
  Vx_FL : Outport
  Vx_FR : Outport  Port=2
  Vx_RL : Outport  Port=3
  Vx_RR : Outport  Port=4
  alpha_FL : Outport  Port=5
  alpha_FR : Outport  Port=6
  alpha_RL : Outport  Port=7
  alpha_RR : Outport  Port=8
  wires:
  <deltaR>/1 -> MATLAB Function2/5(delta_R)
  <deltaL>/1 -> MATLAB Function2/4(delta_L)
  MATLAB Function2/8(alpha_RR) -> alpha_RR/1
  Constant1/1 -> MATLAB Function2/7(b), MATLAB Function2/6(a)
  MATLAB Function2/2(V_FR) -> Vx_FR/1
  MATLAB Function2/1(V_FL) -> Vx_FL/1
  <Vy>/1 -> MATLAB Function2/2(Vy)
  MATLAB Function2/3(V_RL) -> Vx_RL/1
  MATLAB Function2/4(V_RR) -> Vx_RR/1
  MATLAB Function2/5(alpha_FL) -> alpha_FL/1
  <Yaw Rate>/1 -> MATLAB Function2/3(phi_dot)
  MATLAB Function2/7(alpha_RL) -> alpha_RL/1
  <Vx>/1 -> MATLAB Function2/1(Vx)
  Constant2/1 -> MATLAB Function2/8(t)
  MATLAB Function2/6(alpha_FR) -> alpha_FR/1
  Constant/1 -> MATLAB Function2/9(Vx_min)

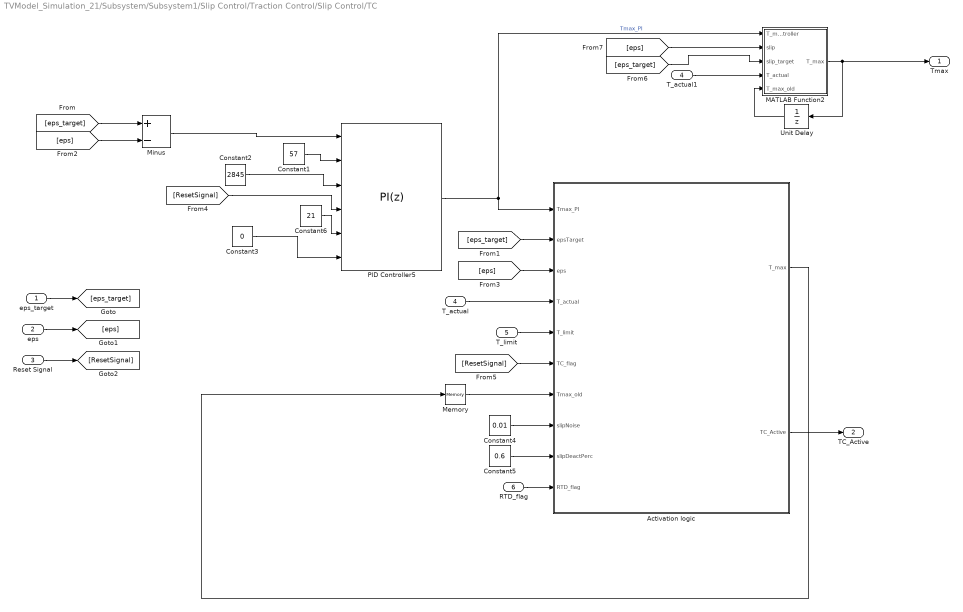
== system TVModel_Simulation_21/Subsystem/Subsystem1/Slip Control/Traction Control/Slip Control/TC ==
  eps_target : Inport
  eps : Inport  Port=2
  Reset Signal : Inport  Port=3
  T_actual : Inport  Port=4  PortDimensions=4
  T_limit : Inport  Port=5
  RTD_flag : Inport  Port=6
  Activation logic : Stateflow chart  TreatAsAtomicUnit=on
  Constant1 : Constant  Value=57
  Constant2 : Constant  Value=2845
  Constant3 : Constant  Value=0
  Constant4 : Constant  Value=0.01
  Constant5 : Constant  Value=0.6
  Constant6 : Constant  Value=21
  MATLAB Function2 : MATLAB Function  TreatAsAtomicUnit=on
  Memory : Memory  InheritSampleTime=on
  Minus : Sum  Inputs=+-
  PID Controller5 : slpidlib/PID Controller  Controller=PI  Form=Parallel  TimeDomain=Discrete-time  UseExternalTs=off  SampleTime=0.02  IntegratorMethod=Forward Euler  FilterMethod=Forward Euler  ControllerParametersSource=external  P=57  I=2845  D=0  UseFilter=off  N=63.8249907657072  TunerSelectOption=Transfer Function Based (PID Tuner App)  InitialConditionSource=internal  InitialConditionForIntegrator=0  InitialConditionForFilter=0  DifferentiatorICPrevScaledInput=0  ExternalReset=rising  TrackingMode=off  Kt=TV_OLD.LV.GEN.slipKt  LimitOutput=on  SatLimitsSource=external  UpperSaturationLimit=21*TV_OLD.CAR.tau  LowerSaturationLimit=5*TV_OLD.CAR.tau  LinearizeAsGain=on  AntiWindupMode=clamping  Kb=1  POutMin=[]  POutMax=[]  IOutMin=[]  IOutMax=[]  DOutMin=[]  DOutMax=[]  NOutMin=[]  NOutMax=[]  SumOutMin=[]  SumOutMax=[]  SaturationOutMin=[]  SaturationOutMax=[]  PParamMin=[]  PParamMax=[]  IParamMin=[]  IParamMax=[]  DParamMin=[]  DParamMax=[]  NParamMin=[]  NParamMax=[]  KbParamMin=[]  KbParamMax=[]  KtParamMin=[]  KtParamMax=[]  KbOutMin=[]  KbOutMax=[]  KtOutMin=[]  KtOutMax=[]  IntegratorOutMin=[]  IntegratorOutMax=[]  FilterOutMin=[]  FilterOutMax=[]  SumI1OutMin=[]  SumI1OutMax=[]  SumI2OutMin=[]  SumI2OutMax=[]  SumI3OutMin=[]  SumI3OutMax=[]  SumI4OutMin=[]  SumI4OutMax=[]  SumDOutMin=[]  SumDOutMax=[]  DifferentiatorOutMin=[]  DifferentiatorOutMax=[]  FilterDiffOutCoefMin=[]  FilterDiffOutCoefMax=[]  ReciprocalOutMin=[]  ReciprocalOutMax=[]  SumDenOutMin=[]  SumDenOutMax=[]  SumNumOutMin=[]  SumNumOutMax=[]  DivideOutMin=[]  DivideOutMax=[]  UdiffTsProdOutMin=[]  UdiffTsProdOutMax=[]  NTsProdOutMin=[]  NTsProdOutMax=[]  UintegralTsProdOutMin=[]  UintegralTsProdOutMax=[]  UngainTsProdOutMin=[]  UngainTsProdOutMax=[]  IntegratorContinuousStateAttributes=''  IntegratorStateMustResolveToSignalObject=off  IntegratorRTWStateStorageClass=Auto  FilterContinuousStateAttributes=''  FilterStateMustResolveToSignalObject=off  FilterRTWStateStorageClass=Auto  ParallelPVariant=ExternalParameters  IdealPVariant=Disabled  IVariant=ExternalParameters  DVariant=Disabled  IntegratorVariant=Discrete  SatVariant=External  AWVariant=DiscClampingParallel  PCopyVariant=Disabled  TRVariant=Disabled  FdbkBlocksVariant=Forward  IdealPFdbkVariant=Disabled  SatFdbkVariant=Disabled  DerivativeFilterVariant=Disabled  NVariant=Disabled  NCopyVariant=Disabled_SignalSpec  FilterICVariant=Disabled  IntegratorICVariant=InternalICs  ExternalResetVariant=ExternalReset  TRSumVariant=Passthrough  SumFdbkVariant=Disabled  SumVariant=Sum_PI  TsampFilterVariant=InternalTs  TsampNgainVariant=Passthrough  TsampIntegralVariant=Passthrough  ExternalSaturationOutDataTypeStr=Inherit: Same as second input
  T_actual1 : InportShadow  Port=4  PortDimensions=4
  Unit Delay : UnitDelay  SampleTime=-1  HasFrameUpgradeWarning=on
  Tmax : Outport
  TC_Active : Outport  Port=2
  wires:
  [eps_target] -> MATLAB Function2/3(slip_target)
  Unit Delay/1 -> MATLAB Function2/5(T_max_old)
  T_actual1/1 -> MATLAB Function2/4(T_actual)
  [eps] -> MATLAB Function2/2(slip)
  MATLAB Function2/1(T_max) -> Unit Delay/1, Tmax/1
  Constant5/1 -> Activation logic/9(slipDeactPerc)
  Constant6/1 -> PID Controller5/5
  Constant3/1 -> PID Controller5/6
  Constant1/1 -> PID Controller5/2
  [ResetSignal] -> Activation logic/6(TC_flag)
  [ResetSignal] -> PID Controller5/4
  [eps] -> Activation logic/3(eps)
  [eps_target] -> Activation logic/2(epsTarget)
  [eps_target] -> Minus/1
  Reset Signal/1 -> [ResetSignal]
  eps/1 -> [eps]
  eps_target/1 -> [eps_target]
  T_limit/1 -> Activation logic/5(T_limit)
  PID Controller5/1 -> MATLAB Function2/1(T_max_controller), Activation logic/1(Tmax_PI)  "Tmax_PI"
  Memory/1 -> Activation logic/7(Tmax_old)
  [eps] -> Minus/2
  T_actual/1 -> Activation logic/4(T_actual)
  Activation logic/1(T_max) -> Memory/1
  Minus/1 -> PID Controller5/1
  Constant4/1 -> Activation logic/8(slipNoise)
  RTD_flag/1 -> Activation logic/10(RTD_flag)
  Activation logic/2(TC_Active) -> TC_Active/1
  Constant2/1 -> PID Controller5/3

== system TVModel_Simulation_21/Subsystem/Subsystem1/Slip Control/Traction Control/Slip Control/epsTarget computation ==
  alpha wheels : Inport
  Abs : Abs
  Constant : Constant  Value=0.96
  Constant1 : Constant
  Constant4 : Constant
  Minus : Sum  Inputs=+-
  Plus1 : Sum
  Product2 : Product
  Product3 : Product
  kappaTarget selection : Subsystem
  epsTarget : Outport
  wires:
  Product3/1 -> Plus1/1
  Product2/1 -> Plus1/2
  kappaTarget selection/1(kappaTarget) -> Product2/2  "kappaTarget"
  Constant4/1 -> Minus/1
  Constant1/1 -> Product3/1
  Constant/1 -> Minus/2, Product2/1
  Minus/1 -> Product3/2
  Abs/1 -> kappaTarget selection/1(alphaWheel)
  alpha wheels/1 -> Abs/1
  Plus1/1 -> epsTarget/1  "epsTarget"

== system TVModel_Simulation_21/Subsystem/Subsystem1/Slip Control/Traction Control/Slip Control/slip ratio ==
  v_wheels : Inport
  w : Inport  Port=2
  Constant : Constant  Value=3
  Discrete Derivative : simulink/Discrete/Discrete Derivative  gainval=1.0  ICPrevScaledInput=0.0  OutMin=[]  OutMax=[]  OutDataType=fixdt(1, 16)  OutScaling=2^-10  DoSatur=off
  Gain : Gain  Gain=0.235
  Gain2 : Gain  Gain=1/9.81
  MATLAB Function : MATLAB Function  TreatAsAtomicUnit=on
  kappa : Outport
  eta : Outport  Port=2
  wires:
  w/1 -> Gain/1
  Gain/1 -> Discrete Derivative/1, MATLAB Function/2(wR)  "ome_wheels"
  Discrete Derivative/1 -> Gain2/1
  Gain2/1 -> eta/1
  v_wheels/1 -> MATLAB Function/1(vx_wheels)  "v_wheels"
  MATLAB Function/1(k) -> kappa/1  "k_prova"
  Constant/1 -> MATLAB Function/3(vx_min)

== system TVModel_Simulation_21/Subsystem/Subsystem1/Slip Control/Traction Control/TC/Load Transfer Calculation1 ==
  In Bus Element : Inport  PortName=dynamics_data
  Fz FL : Subsystem
  Fz FR : Subsystem
  Fz RL : Subsystem
  Fz RR : Subsystem
  Mux : Mux
  Fz [4x1] : Outport
  wires:
  Mux/1 -> Fz [4x1]/1
  Fz RR/1(TV_Info) -> Mux/4  "Fz_RR"
  Fz RL/1(TV_Info) -> Mux/3  "Fz_RL"
  Fz FR/1(TV_Info) -> Mux/2  "Fz_FR"
  Fz FL/1(TV_Info) -> Mux/1  "Fz_FL"
  In Bus Element/1 -> Fz RR/1(dynamics_data), Fz RL/1(dynamics_data), Fz FR/1(dynamics_data), Fz FL/1(dynamics_data)

== system TVModel_Simulation_21/Subsystem/Subsystem1/Slip Control/Traction Control/TC/Subsystem ==
  Inport : Inport
  Inport1 : Inport  Port=2
  Chart : Stateflow chart  TreatAsAtomicUnit=on
  Chart1 : Stateflow chart  TreatAsAtomicUnit=on
  Chart2 : Stateflow chart  TreatAsAtomicUnit=on
  Chart3 : Stateflow chart  TreatAsAtomicUnit=on
  Demux : Demux
  Demux1 : Demux
  Mux : Mux
  Output : Outport
  wires:
  Chart/1(TC_max) -> Mux/1  "TC_output"
  Chart1/1(TC_max) -> Mux/2  "TC_output"
  Chart2/1(TC_max) -> Mux/3  "TC_output"
  Chart3/1(TC_max) -> Mux/4  "TC_output"
  Mux/1 -> Output/1  "TC_output"
  Inport1/1 -> Demux/1
  Inport/1 -> Demux1/1
  Demux1/1 -> Chart/1(T_ff)
  Demux1/2 -> Chart1/1(T_ff)
  Demux1/3 -> Chart2/1(T_ff)
  Demux1/4 -> Chart3/1(T_ff)
  Demux/4 -> Chart3/2(epsilon)
  Demux/3 -> Chart2/2(epsilon)
  Demux/2 -> Chart1/2(epsilon)
  Demux/1 -> Chart/2(epsilon)

== system TVModel_Simulation_21/Subsystem/Subsystem1/Torque Distribution/MPC/ PRE LUDO/Brake & ESP ==
  ubu_in : Inport
  In Bus Element13 : Inport  Port=2  PortName=brake_signal  Element=regen
  Constant : Constant  Commented=on
  Constant1 : Constant  Commented=on  Value=0
  Product : Product  Commented=on
  Switch : Switch  Commented=on  Criteria=u2 > Threshold  Threshold=0.95
  ubu_out : Outport
  wires:
  Constant/1 -> Switch/3
  Constant1/1 -> Switch/1
  ubu_in/1 -> ubu_out/1
  Switch/1 -> Product/2
  Product/1 -> ?
  In Bus Element13/1 -> Switch/2

== system TVModel_Simulation_21/Subsystem/Subsystem1/Torque Distribution/MPC/ PRE LUDO/Faul Detection ==
  note: Utilizzando Simple Torque OCP Status può andare sempre in OCP 4
  In1 : Inport
  OCP Status : Inport  Port=2
  Action Port : Inport  Port=3
  dynamics_data : Inport  Port=4
  dynamics_data1 : Inport  Port=5
  driver_inputs : Inport  Port=6
  brake_signal : Inport  Port=7
  In8 : Inport  Port=8
  If1 : If  Commented=on  IfExpression=u1 == 1
  MPC : Subsystem  Commented=on  TreatAsAtomicUnit=on
  Merge : Merge  Commented=on
  Selector : Selector  Commented=on  InputPortWidth=7  IndexOptions=Index vector (dialog)  Indices=[4:7]  OutputSizes=1
  Simple torque : Subsystem  Commented=on  TreatAsAtomicUnit=on
  Subsystem : Subsystem  Commented=on
  Terminator : Terminator  Commented=on
  Vectorino : Subsystem  Commented=on  TreatAsAtomicUnit=on
  Out1 : Outport
  wires:
  dynamics_data/1 -> Subsystem/2(dynamics_data)
  If1/1 -> MPC/Action
  In8/1 -> Merge/2
  Selector/1 -> MPC/1(In1)  "Torque"
  If1/2 -> Simple torque/Action
  MPC/1(Out1) -> Merge/1
  Vectorino/1(Output) -> Terminator/1
  Merge/1 -> Out1/1
  Subsystem/1(TV Mode Selection) -> If1/1
  OCP Status/1 -> Subsystem/1(OCP Status)
  In1/1 -> Selector/1
  dynamics_data1/1 -> Vectorino/1(dynamics_data)
  driver_inputs/1 -> Vectorino/2(driver_inputs)
  brake_signal/1 -> Vectorino/3(brake_signal)
  Action Port/1 -> Vectorino/Action

== system TVModel_Simulation_21/Subsystem/Subsystem1/Torque Distribution/MPC/ PRE LUDO/Hydraulic brakes ==
  In1 : Inport
  Brake friction : Gain  Commented=on  Gain=0.8
  Braking Areas : Constant  Commented=on  Value=[TV.CAR.BrkArea_front;TV.CAR.BrkArea_front;TV.CAR.BrkArea_rear;TV.CAR.BrkArea_rear]
  Braking Disk Radii : Constant  Commented=on  Value=[TV.CAR.DiskDiameter_front;TV.CAR.DiskDiameter_front;TV.CAR.DiskDiameter_rear;TV.CAR.DiskDiameter_rear]/2
  Product : Product  Commented=on
  Product1 : Product  Commented=on
  Out1 : Outport
  wires:
  Braking Areas/1 -> Product/2
  In1/1 -> Product/1
  Brake friction/1 -> Product1/1
  Product/1 -> Brake friction/1
  Braking Disk Radii/1 -> Product1/2
  Product1/1 -> Out1/1
